simulink model "example_of_step_block"  (R2021a)
settings: Solver=VariableStepAuto  StartTime=0.0  StopTime=10.0  RelTol=1e-3
settings Model: Creator=YasserNet  LastModifiedBy=YasserNet

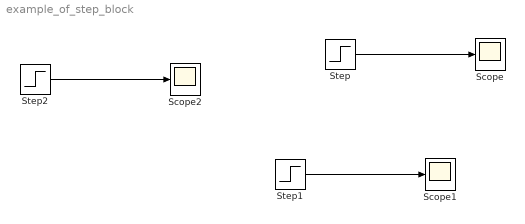
== system example_of_step_block ==
  Scope : Scope
  Scope1 : Scope
  Scope2 : Scope
  Step : Step  Time=0  SampleTime=0
  Step1 : Step  Time=2  SampleTime=0
  Step2 : Step  Time=2  Before=-2  After=5  SampleTime=0
  wires:
  Step/1 -> Scope/1
  Step1/1 -> Scope1/1
  Step2/1 -> Scope2/1
